simulink model "test01_agri"  (R2021a)
settings: Solver=VariableStepAuto  StartTime=0.0  StopTime=10  RelTol=1e-3
libraries: HORTISIM x7
settings Model: Creator=djoroya  LastModifiedBy=djoroya
settings DebuggingCC: UnconnectedInputMsg=none  UnconnectedOutputMsg=none  UnconnectedLineMsg=none

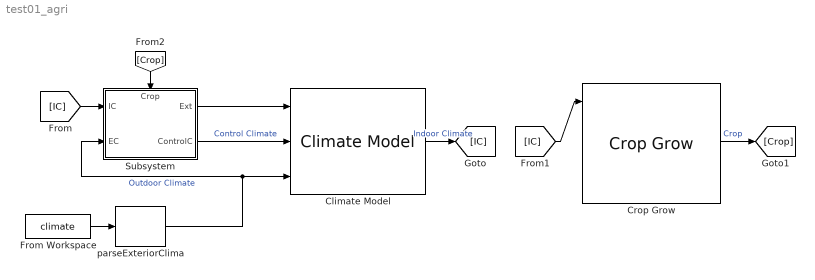
== system test01_agri ==
  Climate Model : HORTISIM/Climate/Models/Climate Model  hour0=0  G0=[0.05 0.0007]  T0=[273 273 273 273]+15  H=7  A_f=3200  A_c=3200  minWindows=0.1  lam_s=[2.5000 0.8500]  c_s=[1081 1081]  l_s=[0.1000 0.1000]  rhod_s=[2600 2500]  int_air_speed=0.5  alpha_i=0.1  alpha_c=0.05  tau_c=0.9  alpha_f=0.1  d_c=1.5  cd_c=8736  T_ss=285.15
      settings: SourceProductName=Horti Simulator
  Crop Grow : HORTISIM/Horticulture/Models/Crop Grow  Chi_nutrients="[ 0.0156    0.0104    0.0052    0.0021    0.0021    0.0010         0         0]"  A_v=2080  plants_density=2.1562  fraction_DM=0.08  min_water_capacity=0.1  C_buf_max=0.02  T_v_start_fruit=1100  int_air_speed=0.5  b_N_uptake=0.5  Tv=288  C=[0.0100 1.0000e-03 0.0100 0.0100]  R=[0 0 0]  Tsum=0  C_wv=0.2  N=zeros(8,1)  rg_fruit=2e-7  c_fruit_m=2.3e-7  c_fruit_g=0.27  rg_leaf=9.5000e-08  c_leaf_m=3.4700e-07  c_leaf_g=0.28  rg_stem=7.4000e-08  c_stem_m=1.47e-7  c_stem_g=0.3  T_max_v=40  s_max_T=0.5793  s_min_T=-0.8690  s_buforg_buf=-5000  T_sum_end=1035  T_max_v24=27  T_min_v24=14  s_min_T24=-1.1587  s_max_T24=1.3904  T_min_v=6
      settings: SourceProductName=Horti Simulator
  From Workspace : FromWorkspace  VariableName=climate
  Subsystem : Subsystem
      settings: PortSchema="{\"entries\":[{\"content\":{\"sides\":[{\"content\":{\"connectorIds\":[\"In1\",\"In2\"]},\"type\":\"ConnectorPlacement.EquallySpacedRectSide\",\"uuid\":\"05a20284-31f0-4954-ac42-b08c051c723b\"},{\"content\":{\"connectorIds\":[\"Out1\",\"Out2\"],\"side\":\"RIGHT\"},\"type\":\"ConnectorPlacement.EquallySpacedRectSide\",\"uuid\":\"7e4ab434-6629-473e-82a5-f81f17f0ab6e\"},{\"content\":{\"connectorIds\":[\"In3\"],\"side\":\"TOP\"},\"type\":\"ConnectorPlacement.EquallySpacedRectSide\",\"uuid\":\"2ea64524-8947-456a-a977-2c05776eabaa\"}]},\"type\":\"ConnectorPlacement.EquallySpacedConnector\",\"uuid\":\"6035ded9-300f-4f3c-adde-f9d2e7ea6cf9\"}],\"packageUris\":[\"http://schema.mathworks.com/mf0/Connector/R2020b\"],\"version\":\"1.0\"}"
  parseExteriorClima : HORTISIM/Other  Functions/parseExteriorClima  SystemSampleTime=-1  VariantActivationTime=update diagram  Latency=0  AutoFrameSizeCalculation=off
      settings: SourceProductName=Horti Simulator
  wires:
  From Workspace/1 -> parseExteriorClima/1
  parseExteriorClima/1 -> Climate Model/3, Subsystem/2(EC)  "Outdoor Climate"
  Climate Model/1 -> [IC]  "Indoor Climate"
  Subsystem/2(ControlC) -> Climate Model/2  "Control Climate"
  [IC] -> Subsystem/1(IC)
  Subsystem/1(Ext) -> Climate Model/1
  [IC] -> Crop Grow/1
  Crop Grow/1 -> [Crop]  "Crop"
  [Crop] -> Subsystem/3(Crop)

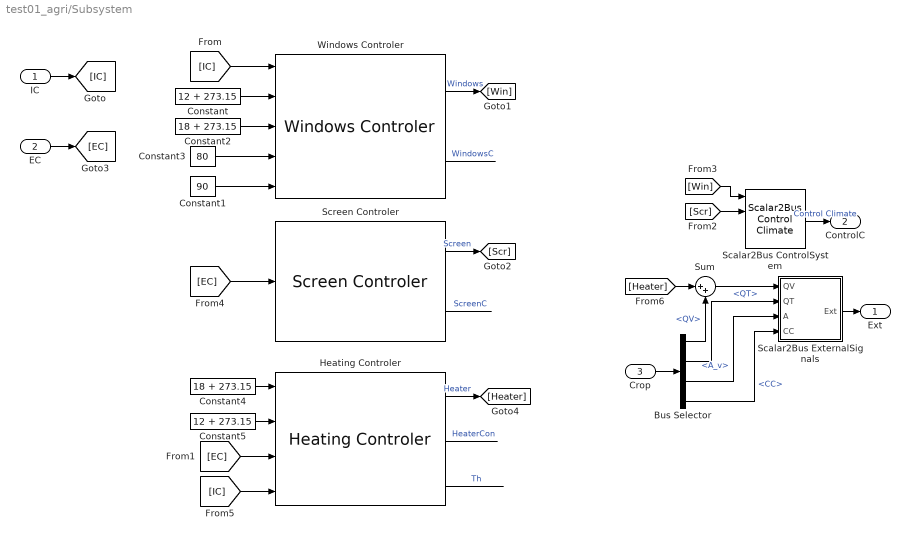
== system test01_agri/Subsystem ==
  IC : Inport
  EC : Inport  Port=2
  Crop : Inport  Port=3
  Bus Selector : BusSelector  OutputSignals=HeatVars.QV,HeatVars.QT,A_v,CC
  Constant : Constant  Value=12 + 273.15
  Constant1 : Constant  Value=90
  Constant2 : Constant  Value=18 + 273.15
  Constant3 : Constant  Value=80
  Constant4 : Constant  Value=18 + 273.15
  Constant5 : Constant  Value=12 + 273.15
  Heating Controler : HORTISIM/Climate/Controls/Heating Controler  T=288  power=1000e3  A_e=6e-4  A_i=6e-4  c=1e-8
      settings: SourceProductName=Horti Simulator
  Scalar2Bus ControlSystem : HORTISIM/Other  Functions/Scalar2Bus  Control Climate  SystemSampleTime=-1  VariantActivationTime=update diagram  Latency=0  AutoFrameSizeCalculation=off
      settings: SourceProductName=Horti Simulator
  Scalar2Bus ExternalSignals : Subsystem
  Screen Controler : HORTISIM/Climate/Controls/Screen Controler  Radthreshold=200  velocity=0.33333  Power=0  gamma_max=0.3  beta=0.1
      settings: SourceProductName=Horti Simulator
  Sum : Sum  Inputs=|++
  Windows Controler : HORTISIM/Climate/Controls/Windows Controler  Power=100  max_night=10  tau=600  RadThreshold=10  AR=10
      settings: SourceProductName=Horti Simulator
  Ext : Outport
  ControlC : Outport  Port=2
  wires:
  Constant2/1 -> Windows Controler/3
  Constant3/1 -> Windows Controler/4
  Windows Controler/2 -> ?  "WindowsC"
  Constant1/1 -> Windows Controler/5
  Constant/1 -> Windows Controler/2
  IC/1 -> [IC]
  [IC] -> Windows Controler/1
  Windows Controler/1 -> [Win]  "Windows"
  Screen Controler/1 -> [Scr]  "Screen"
  [Scr] -> Scalar2Bus ControlSystem/2
  [Win] -> Scalar2Bus ControlSystem/1
  Scalar2Bus ControlSystem/1 -> ControlC/1  "Control Climate"
  EC/1 -> [EC]
  [EC] -> Screen Controler/1
  Screen Controler/2 -> ?  "ScreenC"
  [EC] -> Heating Controler/3
  [IC] -> Heating Controler/4
  Constant4/1 -> Heating Controler/1
  Constant5/1 -> Heating Controler/2
  Heating Controler/1 -> [Heater]  "Heater"
  Scalar2Bus ExternalSignals/1(Ext) -> Ext/1
  Heating Controler/3 -> ?  "Th"
  Heating Controler/2 -> ?  "HeaterCon"
  Crop/1 -> Bus Selector/1
  Bus Selector/2 -> Scalar2Bus ExternalSignals/2(QT)  "<QT>"
  [Heater] -> Sum/1
  Sum/1 -> Scalar2Bus ExternalSignals/1(QV)
  Bus Selector/1 -> Sum/2  "<QV>"
  Bus Selector/3 -> Scalar2Bus ExternalSignals/3(A)  "<A_v>"
  Bus Selector/4 -> Scalar2Bus ExternalSignals/4(CC)  "<CC>"

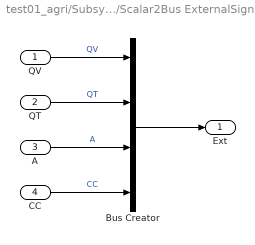
== system test01_agri/Subsystem/Scalar2Bus ExternalSignals ==
  QV : Inport
  QT : Inport  Port=2
  A : Inport  Port=3
  CC : Inport  Port=4
  Bus Creator : BusCreator  Inputs=4
  Ext : Outport
  wires:
  QT/1 -> Bus Creator/2  "QT"
  QV/1 -> Bus Creator/1  "QV"
  A/1 -> Bus Creator/3  "A"
  CC/1 -> Bus Creator/4  "CC"
  Bus Creator/1 -> Ext/1
